simulink model "VTOL_sim_8_f"  (R2018a)
settings: Solver=VariableStepAuto  StartTime=0.0  StopTime=40  RelTol=1e-3
InitFcn:
  | vtol_param
StartFcn:
  | vtol_param
values from neighbouring files (symbols this model uses):
  F = 10    [FT2_Check.m]
  T = 1    [FT2_Check.m]
undefined symbols (not defined in the file or in its folder): FT2fl, FT2fr, P, PlotVtol
ContinueFcn:
  | FT2frfl
settings Model: Creator=sadam  LastModifiedBy=sadam

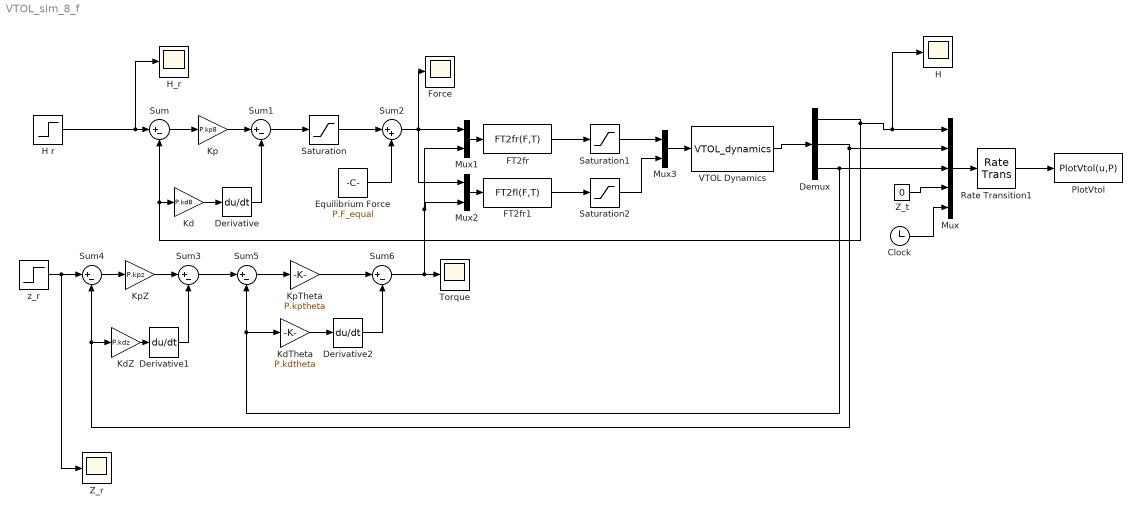
== system VTOL_sim_8_f ==
  Clock : Clock
  Demux : Demux  Outputs=3
  Derivative : Derivative
  Derivative1 : Derivative
  Derivative2 : Derivative
  Equilibrium Force : Constant  Value=P.F_equal
  FT2fr : MATLABFcn  MATLABFcn=FT2fr(F,T)  OutputSignalType=real
  FT2fr1 : MATLABFcn  MATLABFcn=FT2fl(F,T)  OutputSignalType=real
  Force : Scope
  H : Scope
  H r : Step  Time=0  After=5  SampleTime=0
  H_r : Scope
  Kd : Gain  Gain=P.kd8
  "KdTheta " : Gain  Gain=P.kdtheta
  "KdZ " : Gain  Gain=P.kdz
  Kp : Gain  Gain=P.kp8
  "KpTheta " : Gain  Gain=P.kptheta
  "KpZ " : Gain  Gain=P.kpz
  Mux : Mux  Inputs=5
  Mux1 : Mux  Inputs=2
  Mux2 : Mux  Inputs=2
  Mux3 : Mux  Inputs=2
  "PlotVtol " : MATLABFcn  MATLABFcn=PlotVtol(u,P)  OutputDimensions=0
  Rate Transition1 : RateTransition  OutPortSampleTime=P.t_plot
  Saturation : Saturate  UpperLimit=P.Force_max  LowerLimit=-P.Force_max
  Saturation1 : Saturate  UpperLimit=P.Force_max  LowerLimit=-P.Force_max
  Saturation2 : Saturate  UpperLimit=P.Force_max  LowerLimit=-P.Force_max
  Sum{,1,3..6} (6 alike) : Sum  Inputs=|+-
  Sum2 : Sum  Inputs=|++
  Torque : Scope
  VTOL Dynamics : S-Function  FunctionName=VTOL_dynamics  Parameters=P  SFunctionDeploymentMode=off  EnableBusSupport=off
  "Z_r " : Scope
  Z_t : Constant  Value=0
  "z_r " : Step  Time=10  After=0  SampleTime=0
  wires:
  Sum/1 -> Kp/1
  Kd/1 -> Derivative/1
  Kp/1 -> Sum1/1
  Derivative/1 -> Sum1/2
  Mux/1 -> Rate Transition1/1
  VTOL Dynamics/1 -> Demux/1
  Saturation/1 -> Sum2/1
  Equilibrium Force/1 -> Sum2/2
  Sum1/1 -> Saturation/1
  Rate Transition1/1 -> "PlotVtol "/1
  Z_t/1 -> Mux/4
  Clock/1 -> Mux/5
  "KpZ "/1 -> Sum3/1
  Sum4/1 -> "KpZ "/1
  Sum3/1 -> Sum5/1
  "KdZ "/1 -> Derivative1/1
  Derivative1/1 -> Sum3/2
  Sum5/1 -> "KpTheta "/1
  "KdTheta "/1 -> Derivative2/1
  "KpTheta "/1 -> Sum6/1
  Derivative2/1 -> Sum6/2
  Demux/1 -> H/1, Mux/1, Kd/1, Sum/2
  Sum2/1 -> Mux2/1, Mux1/1, Force/1
  Sum6/1 -> Torque/1, Mux2/2, Mux1/2
  H r/1 -> H_r/1, Sum/1
  Demux/2 -> "KdZ "/1, Sum4/2, Mux/2
  Demux/3 -> "KdTheta "/1, Sum5/2, Mux/3
  Mux1/1 -> FT2fr/1
  Mux2/1 -> FT2fr1/1
  Mux3/1 -> VTOL Dynamics/1
  "z_r "/1 -> "Z_r "/1, Sum4/1
  Saturation1/1 -> Mux3/1
  FT2fr/1 -> Saturation1/1
  Saturation2/1 -> Mux3/2
  FT2fr1/1 -> Saturation2/1
